simulink model "coupled_tanks_quick_start"  (R2015a)
settings: Solver=ode1  StartTime=0.0  StopTime=inf  FixedStep=0.002  RelTol=1e-3
PostLoadFcn:
  | qc_set_target_type(getConfigSet(bdroot, 'QUARC Default Target Configuration'));
settings Model: SimulationMode=external  CovSFcnEnable=off  ExtModeTrigDuration=30000  Creator=MLevis  LastModifiedBy=Aluno IC
settings SolverCC: PositivePriorityOrder=on
settings DataIOCC: SignalLoggingSaveFormat=ModelDataLogs
settings OptimizationCC: ExpressionDepthLimit=2147483647  InitFltsAndDblsToZero=on
settings DebuggingCC: SaveWithParameterizedLinksMsg=none  UnderspecifiedInitializationDetection=Classic  MergeDetectMultiDrivingBlocksExec=none  SolverPrmCheckMsg=warning  MultiTaskDSMMsg=warning  MultiTaskCondExecSysMsg=none  FcnCallInpInsideContextMsg=UseLocalSettings  StateNameClashWarn=warning
settings RTWCC: SystemTargetFile=quarc_win64.tlc  TemplateMakefile=quarc_default_tmf  Description=QUARC Win64 Target
settings STFCustomTargetCC: TargetLibSuffix=.lib  TargetPreCompLibLocation=C:\PROGRA~3\QUARC\lib\2014a\win64\release  GenerateSampleERTMain=off  ConcurrentExecutionCompliant=on  GeneratePreprocessorConditionals=Disable all  ERTCustomFileBanners=off  SupportNonInlinedSFcns=on  SupportVariableSizeSignals=off  MATLABClassNameForMDSCustomization=Simulink.SoftwareTarget.GRTCustomization  CPPClassGenCompliant=on  GRTInterface=on  SystemTargetFile=quarc_win64.tlc
settings GRTTargetCC: TargetPreCompLibLocation=C:\PROGRA~3\QUARC\lib\2014a\win64\release  ParMdlRefBuildCompliant=off  CompOptLevelCompliant=off  CombineOutputUpdateFcns=off  MatFileLogging=off  GRTInterface=on  ExtMode=on  ExtModeMexFile=quarc_comm

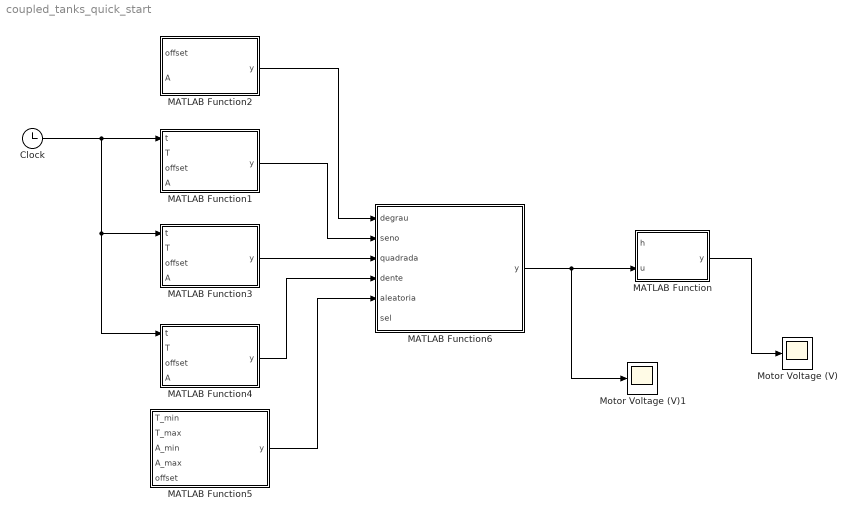
== system coupled_tanks_quick_start ==
  Clock : Clock
  MATLAB Function : MATLAB Function  TreatAsAtomicUnit=on
  MATLAB Function1 : MATLAB Function  TreatAsAtomicUnit=on
  MATLAB Function2 : MATLAB Function  TreatAsAtomicUnit=on
  MATLAB Function3 : MATLAB Function  TreatAsAtomicUnit=on
  MATLAB Function4 : MATLAB Function  TreatAsAtomicUnit=on
  MATLAB Function5 : MATLAB Function  TreatAsAtomicUnit=on
  MATLAB Function6 : MATLAB Function  TreatAsAtomicUnit=on
  Motor Voltage (V) : Scope
      settings: TimeRange=30  YMin=0  YMax=25
  Motor Voltage (V)1 : Scope
      settings: TimeRange=30  YMin=0  YMax=25  SaveName=ScopeData3
  wires:
  Clock/1 -> MATLAB Function4/1(t), MATLAB Function3/1(t), MATLAB Function1/1(t)
  MATLAB Function2/1(y) -> MATLAB Function6/1(degrau)
  MATLAB Function1/1(y) -> MATLAB Function6/2(seno)
  MATLAB Function3/1(y) -> MATLAB Function6/3(quadrada)
  MATLAB Function4/1(y) -> MATLAB Function6/4(dente)
  MATLAB Function5/1(y) -> MATLAB Function6/5(aleatoria)
  MATLAB Function/1(y) -> Motor Voltage (V)/1
  MATLAB Function6/1(y) -> Motor Voltage (V)1/1, MATLAB Function/2(u)

== matlab function coupled_tanks_quick_start/MATLAB Function1 ==
  data: t input; y output; T input; offset input; A input
function y = seno(t, T, offset, A)

y = A*sin(t*2*pi/T) + offset;

== matlab function coupled_tanks_quick_start/MATLAB Function ==
  data: h input; u input; y output
function y = fcn(h, u)
%#codegen
h_max = 30;

%Trava de tensão
if(u < -4)
    u = -4;
end
if(u > 4)
    u = 4;
end

%Trava pra não sugar ar
if(u < 0 & h < 2)
    u = 0;
end

%Trava de transbordamento
if(h >= h_max - 1.0  & h < h_max - 0.75)
    u = 0.95*u;
elseif(h >= h_max - 0.75 & h < h_max - 0.5)
    u = 0.93*u;
elseif(h >= h_max - 0.5 & h < h_max - 0.25)
    u = 0.91*u;
elseif(h >= h_max - 0.25 & h < h_max)
    u = 0.88*u;
elseif(h >= h_max)
    u = 0;
end
    
y = u;

== matlab function coupled_tanks_quick_start/MATLAB Function2 ==
  data: y output; offset input; A input
function y = degrau(offset, A)

y = A + offset;

== matlab function coupled_tanks_quick_start/MATLAB Function3 ==
  data: t input; y output; T input; offset input; A input
function y = quadrada(t, T, offset, A)

y = A*square(t*2*pi/T) + offset;

== matlab function coupled_tanks_quick_start/MATLAB Function4 ==
  data: t input; y output; T input; offset input; A input
function y = dente(t, T, offset, A)

y = A*sawtooth(t*2*pi/T) + offset;

== matlab function coupled_tanks_quick_start/MATLAB Function5 ==
  data: T_min input; y output; T_max input; A_min input; A_max input; offset input
function y = aleatoria(T_min, T_max, A_min, A_max, offset)

T_now = T_min + (T_max - T_min)*rand;
A_now = A_min + (A_max - A_min)*rand + offset;

pause(T_now)

y = A_now;

== matlab function coupled_tanks_quick_start/MATLAB Function6 ==
  data: degrau input; y output; seno input; quadrada input; dente input; aleatoria input; sel input
function y = mux(degrau, seno, quadrada, dente, aleatoria, sel)

switch sel
    case 1
        y = seno;
    case 2
        y = degrau;
    case 3
        y = dente;
    case 4
        y = quadrada;
    case 5
        y = aleatoria;
end
